simulink model "hw481pendulum"  (Simulink 7.0)
settings: Solver=ode45  StartTime=0.0  StopTime=20  FixedStep=Tsample  RelTol=1e-5
settings Model: Creator=Kostas Tsakalis  LastModifiedBy=KST  ExtModeArmWhenConnect=off  BufferReuse=off
settings DataIOCC: LimitDataPoints=off  SaveState=on  OutputSaveName=theta  SignalLoggingName=sigsOut
settings OptimizationCC: BlockReduction=off  OptimizeBlockIOStorage=off  BufferReuse=off  EnforceIntegerDowncast=off  ExpressionFolding=off  FoldNonRolledExpr=off  LocalBlockOutputs=off
settings DebuggingCC: SaveWithParameterizedLinksMsg=none  SignalResolutionControl=TryResolveAllWithWarning  SolverPrmCheckMsg=none  MultiTaskDSMMsg=warning  MultiTaskCondExecSysMsg=none  StrictBusMsg=None
settings HardwareCC: TargetEndianess=LittleEndian  TargetHWDeviceType=MATLAB Host  ProdEqTarget=off
settings RTWCC: SystemTargetFile=xpctarget.tlc  TemplateMakefile=xpc_default_tmf  Description=xPC Target  ProcessScript=xpctarget_make_rtw_hook  IncludeERTFirstTime=on
settings xpcTargetCC: TargetFcnLib=ansi_tfl_tmw.mat  GenFloatMathFcnCalls=ANSI_C  CompOptLevelCompliant=off  PortableWordSizes=off

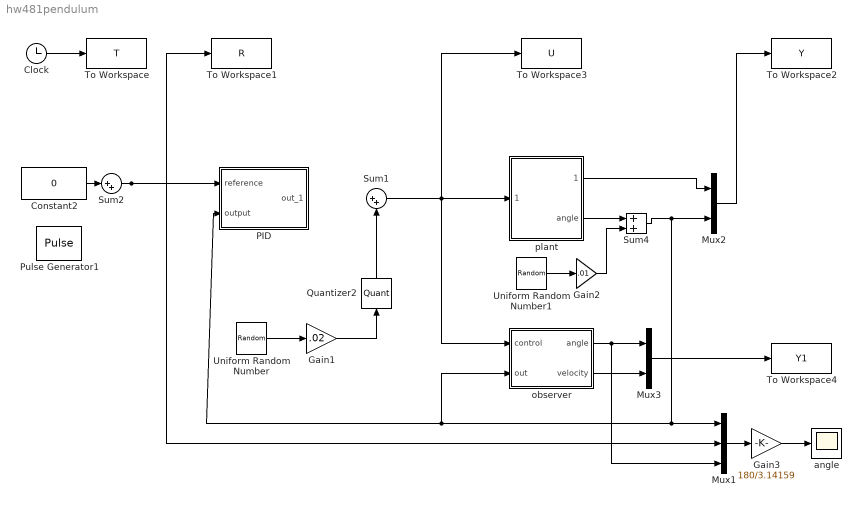
== system hw481pendulum ==
  Clock : Clock
      settings: Decimation=10
  Constant2 : Constant  Value=0  OutDataType=sfix(16)  OutScaling=2^0
  Gain1 : Gain  Gain=.02  ParameterDataType=sfix(16)  ParameterScaling=2^0  OutDataType=sfix(16)  OutScaling=2^0  SaturateOnIntegerOverflow=on
  Gain2 : Gain  Gain=.01  ParameterDataType=sfix(16)  ParameterScaling=2^0  OutDataType=sfix(16)  OutScaling=2^0  SaturateOnIntegerOverflow=on
  Gain3 : Gain  Gain=180/3.14159  ParameterDataType=sfix(16)  ParameterScaling=2^0  OutDataType=sfix(16)  OutScaling=2^0  SaturateOnIntegerOverflow=on
  Mux1 : Mux  Inputs=3
  Mux2 : Mux  Inputs=2
  Mux3 : Mux  Inputs=2
  PID : Subsystem
  Pulse Generator1 : DiscretePulseGenerator  PulseType=Time based  Amplitude=.2  Period=4  PulseWidth=50  PhaseDelay=1
  Quantizer2 : Quantizer  Orientation=up  QuantizationInterval=2/(2^10)
  Sum1 : Sum  Inputs=|++  OutDataType=sfix(16)  OutScaling=2^0  SaturateOnIntegerOverflow=on
  Sum2 : Sum  Inputs=|++  OutDataType=sfix(16)  OutScaling=2^0  SaturateOnIntegerOverflow=on
  Sum4 : Sum  Inputs=2  OutDataType=sfix(16)  OutScaling=2^0  SaturateOnIntegerOverflow=on
  To Workspace : ToWorkspace  VariableName=T  SampleTime=.01  SaveFormat=Array
  To Workspace1 : ToWorkspace  VariableName=R  SampleTime=.01  SaveFormat=Array
  To Workspace2 : ToWorkspace  VariableName=Y  SampleTime=.01  SaveFormat=Array
  To Workspace3 : ToWorkspace  VariableName=U  SampleTime=.01  SaveFormat=Array
  To Workspace4 : ToWorkspace  VariableName=Y1  SampleTime=.01  SaveFormat=Array
  Uniform Random Number : UniformRandomNumber  SampleTime=.1
  Uniform Random Number1 : UniformRandomNumber  SampleTime=.01
  angle : Scope
      settings: TickLabels=on  TimeRange=20  YMax=15  DataFormat=Array  MaxDataPoints=10000
  observer : Subsystem
  plant : Subsystem  mask{mass=0.2, length=0.5, friction=0, quant=360/(2^12), Sa=1, inquant=2/(2^10), IC=[0 0]}
      mask prompts: quant "quantization"; Sa "saturation (+/-)"; inquant "input quantization"; IC "Initial Conditions (2x1)"
      mask Display: disp('Pendulum \n model')
  wires:
  Constant2/1 -> Sum2/1
  Sum2/1 -> Mux1/2, To Workspace1/1, PID/1(reference)
  plant/2(angle) -> Sum4/1
  Gain3/1 -> angle/1
  Mux1/1 -> Gain3/1
  Clock/1 -> To Workspace/1
  Mux2/1 -> To Workspace2/1
  plant/1(velocity) -> Mux2/1
  Sum1/1 -> plant/1(control), To Workspace3/1, observer/1(control)
  Uniform Random Number/1 -> Gain1/1
  observer/1(angle) -> Mux3/1, Mux1/3
  observer/2(velocity) -> Mux3/2
  Mux3/1 -> To Workspace4/1
  Sum4/1 -> Mux1/1, PID/2(output), observer/2(out), Mux2/2
  Uniform Random Number1/1 -> Gain2/1
  Gain1/1 -> Quantizer2/1
  Quantizer2/1 -> Sum1/2
  Gain2/1 -> Sum4/2

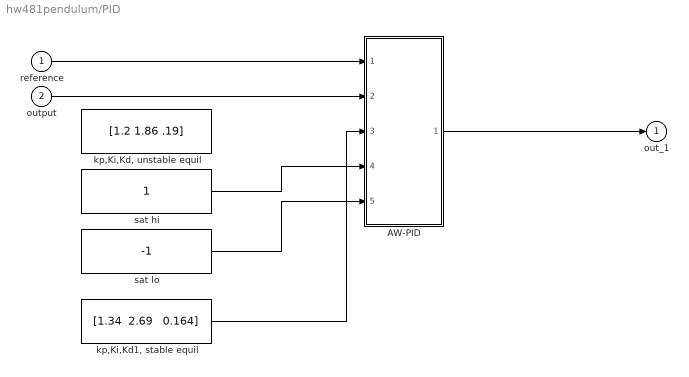
== system hw481pendulum/PID ==
  reference : Inport  OutDataType=sfix(16)  OutScaling=2^0
  output : Inport  Port=2  OutDataType=sfix(16)  OutScaling=2^0
  "AW-PID " : Subsystem  mask(Anti-windup PID ){tau=.005, DT=0.01}
      mask prompts: tau "Pseudo-derivative filter time constant (tustin)"; DT "Reference prefilter [num,den] time constants"
      mask help: Discrete PID with Anti-windup and prefilter
      mask init:
      | t_z=@2(1);t_p=@2(2);
      mask Display: disp('Adaptive\n AW-PID\n+filter')
  "kp,Ki,Kd, unstable equil" : Constant  Value=[1.2 1.86 .19]  OutDataType=sfix(16)  OutScaling=2^0  SampleTime=.01
  "kp,Ki,Kd1, stable equil" : Constant  Value="[1.34  2.69   0.164]"  OutDataType=sfix(16)  OutScaling=2^0  SampleTime=.01
  sat hi : Constant  OutDataType=sfix(16)  OutScaling=2^0
  sat lo : Constant  Value=-1  OutDataType=sfix(16)  OutScaling=2^0
  out_1 : Outport  InitialOutput=0
  wires:
  sat lo/1 -> "AW-PID "/5(input constraint lo)
  sat hi/1 -> "AW-PID "/4(input constraint hi)
  output/1 -> "AW-PID "/2(System Output)
  "AW-PID "/1(Input to system) -> out_1/1
  reference/1 -> "AW-PID "/1(Set point)
  "kp,Ki,Kd1, stable equil"/1 -> "AW-PID "/3(parameters)

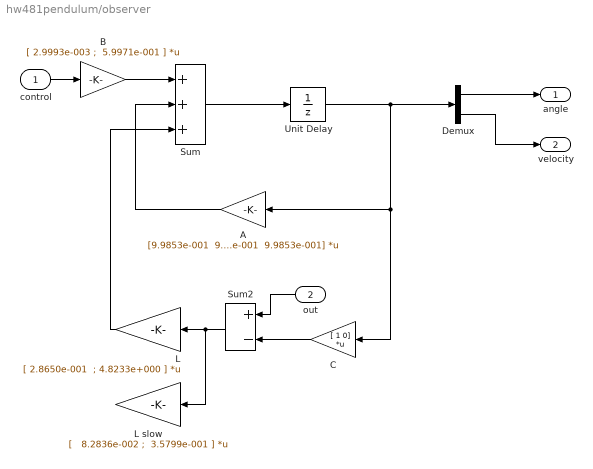
== system hw481pendulum/observer ==
  control : Inport  OutDataType=sfix(16)  OutScaling=2^0
  out : Inport  Orientation=left  Port=2  OutDataType=sfix(16)  OutScaling=2^0
  A : Gain  Orientation=left  Gain=|  Multiplication=Matrix(K*u)  ParameterDataType=sfix(16)  ParameterScaling=2^0  OutDataType=sfix(16)  OutScaling=2^0  SaturateOnIntegerOverflow=on
      | [9.9853e-001  9.9951e-003
      | ; -2.9416e-001  9.9853e-001]
  B : Gain  Gain=|  Multiplication=Matrix(K*u)  ParameterDataType=sfix(16)  ParameterScaling=2^0  OutDataType=sfix(16)  OutScaling=2^0  SaturateOnIntegerOverflow=on
      | [ 2.9993e-003;  5.9971e-001
      | ]
  C : Gain  Orientation=left  Gain="[  1     0]"  Multiplication=Matrix(K*u)  ParameterDataType=sfix(16)  ParameterScaling=2^0  OutDataType=sfix(16)  OutScaling=2^0  SaturateOnIntegerOverflow=on
  Demux : Demux  Outputs=2
  L : Gain  Orientation=left  Gain=|  Multiplication=Matrix(K*u)  ParameterDataType=sfix(16)  ParameterScaling=2^0  OutDataType=sfix(16)  OutScaling=2^0  SaturateOnIntegerOverflow=on
      | [ 2.8650e-001
      |  ; 4.8233e+000
      | ]
  L slow : Gain  Orientation=left  Gain=|  Multiplication=Matrix(K*u)  ParameterDataType=sfix(16)  ParameterScaling=2^0  OutDataType=sfix(16)  OutScaling=2^0  SaturateOnIntegerOverflow=on
      | [   8.2836e-002
      | ;  3.5799e-001
      | ]
  Sum : Sum  Inputs=+++  OutDataType=sfix(16)  OutScaling=2^0  SaturateOnIntegerOverflow=on  InputSameDT=on
  Sum2 : Sum  Orientation=left  Inputs=+-  OutDataType=sfix(16)  OutScaling=2^0  SaturateOnIntegerOverflow=on  InputSameDT=on
  Unit Delay : UnitDelay  SampleTime=.01
  angle : Outport  InitialOutput=0
  velocity : Outport  Port=2  InitialOutput=0
  wires:
  Sum2/1 -> L/1, L slow/1
  out/1 -> Sum2/1
  control/1 -> B/1
  Sum/1 -> Unit Delay/1
  Unit Delay/1 -> Demux/1, A/1, C/1
  Demux/1 -> angle/1
  Demux/2 -> velocity/1
  A/1 -> Sum/2
  B/1 -> Sum/1
  C/1 -> Sum2/2
  L/1 -> Sum/3

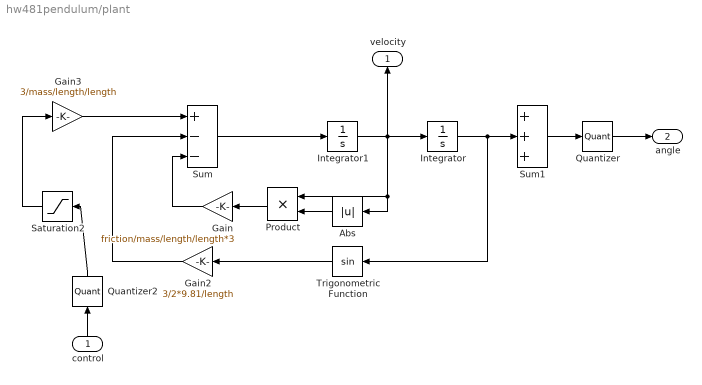
== system hw481pendulum/plant ==
  control : Inport  Orientation=up  OutDataType=sfix(16)  OutScaling=2^0
  Abs : Abs  Orientation=left  OutDataType=sfix(16)  OutScaling=2^0
  Gain : Gain  Orientation=left  Gain=friction/mass/length/length*3  ParameterDataType=sfix(16)  ParameterScaling=2^0  OutDataType=sfix(16)  OutScaling=2^0  SaturateOnIntegerOverflow=on
  Gain2 : Gain  Orientation=left  Gain=3/2*9.81/length  ParameterDataType=sfix(16)  ParameterScaling=2^0  OutDataType=sfix(16)  OutScaling=2^0  SaturateOnIntegerOverflow=on
  Gain3 : Gain  Gain=3/mass/length/length  ParameterDataType=sfix(16)  ParameterScaling=2^0  OutDataType=sfix(16)  OutScaling=2^0  SaturateOnIntegerOverflow=on
  Integrator : Integrator  InitialCondition=IC(1)
  Integrator1 : Integrator  InitialCondition=IC(2)
  Product : Product  Orientation=left  OutDataType=sfix(16)  OutScaling=2^0  RndMeth=Zero
  Quantizer : Quantizer  QuantizationInterval=quant*pi/180
  Quantizer2 : Quantizer  Orientation=up  QuantizationInterval=inquant
  Saturation2 : Saturate  Orientation=left  UpperLimit=Sa  LowerLimit=-Sa
  Sum : Sum  Inputs=+--  OutDataType=sfix(16)  OutScaling=2^0  SaturateOnIntegerOverflow=on  InputSameDT=on
  Sum1 : Sum  Inputs=+++  OutDataType=sfix(16)  OutScaling=2^0  SaturateOnIntegerOverflow=on  InputSameDT=on
  Trigonometric Function : Trigonometry  Orientation=left
  velocity : Outport  Orientation=up  InitialOutput=0
  angle : Outport  Port=2  InitialOutput=0
  wires:
  Quantizer/1 -> angle/1
  Sum1/1 -> Quantizer/1
  control/1 -> Quantizer2/1
  Gain3/1 -> Sum/1
  Gain2/1 -> Sum/2
  Integrator/1 -> Sum1/2, Trigonometric Function/1
  Gain/1 -> Sum/3
  Integrator1/1 -> Integrator/1, velocity/1, Product/1, Abs/1
  Saturation2/1 -> Gain3/1
  Trigonometric Function/1 -> Gain2/1
  Sum/1 -> Integrator1/1
  Product/1 -> Gain/1
  Abs/1 -> Product/2
  Quantizer2/1 -> Saturation2/1

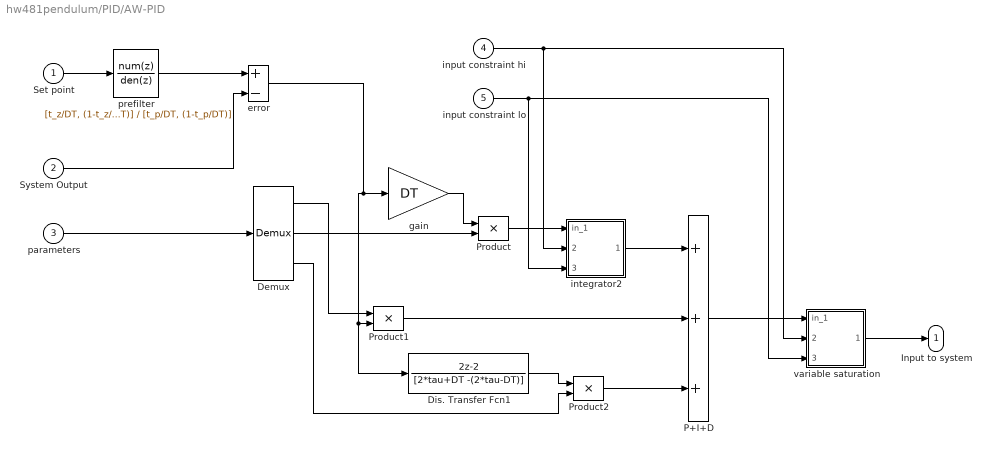
== system hw481pendulum/PID/AW-PID  ==
  Set point : Inport  OutDataType=sfix(16)  OutScaling=2^0
  System Output : Inport  Port=2  OutDataType=sfix(16)  OutScaling=2^0
  parameters : Inport  Port=3  OutDataType=sfix(16)  OutScaling=2^0
  input constraint hi : Inport  Port=4  OutDataType=sfix(16)  OutScaling=2^0
  input constraint lo : Inport  Port=5  OutDataType=sfix(16)  OutScaling=2^0
  Demux : Demux  Outputs=3
  Dis. Transfer Fcn1 : DiscreteTransferFcn  Numerator=[2 -2]  Denominator=[2*tau+DT -(2*tau-DT)]  SampleTime=DT
  P+I+D : Sum  Inputs=+++  OutDataType=sfix(16)  OutScaling=2^0  SaturateOnIntegerOverflow=on  InputSameDT=on
  Product : Product  OutDataType=sfix(16)  OutScaling=2^0  SaturateOnIntegerOverflow=on  InputSameDT=on
  Product1 : Product  OutDataType=sfix(16)  OutScaling=2^0  SaturateOnIntegerOverflow=on  InputSameDT=on
  Product2 : Product  OutDataType=sfix(16)  OutScaling=2^0  SaturateOnIntegerOverflow=on  InputSameDT=on
  error : Sum  Inputs=+-  OutDataType=sfix(16)  OutScaling=2^0  SaturateOnIntegerOverflow=on  InputSameDT=on
  gain : Gain  Gain=DT  ParameterDataType=sfix(16)  ParameterScaling=2^0  OutDataType=sfix(16)  OutScaling=2^0  SaturateOnIntegerOverflow=on
  integrator2 : Subsystem  mask(Anti windup intgrator){DT=DT}
      mask prompts: DT "sampling time"
      mask help: Integral with anti-windup
      mask Display: disp('DT-I-AW')
  prefilter : DiscreteTransferFcn  Numerator=[t_z/DT, (1-t_z/DT)]  Denominator=[t_p/DT, (1-t_p/DT)]  SampleTime=DT
  variable saturation : Subsystem  mask(Anti windup intgrator){DT=DT}
      mask prompts: DT "sampling time"
      mask help: Integral with anti-windup
      mask Display: disp('DT-I-AW')
  Input to system : Outport  InitialOutput=0
  wires:
  input constraint hi/1 -> variable saturation/2(umax), integrator2/2(umax)
  input constraint lo/1 -> variable saturation/3(umin), integrator2/3(umin)
  variable saturation/1(out_1) -> Input to system/1
  System Output/1 -> error/2
  Demux/3 -> Product2/2
  Dis. Transfer Fcn1/1 -> Product2/1
  Product2/1 -> P+I+D/3
  Demux/2 -> Product/2
  Demux/1 -> Product1/1
  gain/1 -> Product/1
  Product/1 -> integrator2/1(in_1)
  P+I+D/1 -> variable saturation/1(in_1)
  integrator2/1(out_1) -> P+I+D/1
  parameters/1 -> Demux/1
  Set point/1 -> prefilter/1
  Product1/1 -> P+I+D/2
  error/1 -> gain/1, Product1/2, Dis. Transfer Fcn1/1
  prefilter/1 -> error/1

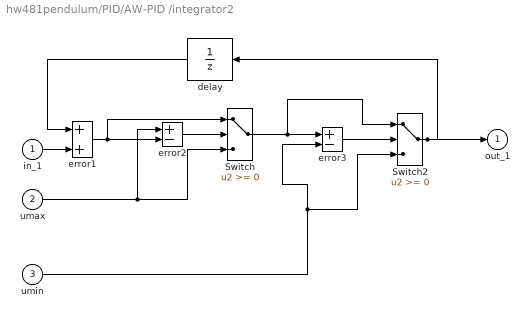
== system hw481pendulum/PID/AW-PID /integrator2 ==
  in_1 : Inport  OutDataType=sfix(16)  OutScaling=2^0
  umax : Inport  Port=2  OutDataType=sfix(16)  OutScaling=2^0
  umin : Inport  Port=3  OutDataType=sfix(16)  OutScaling=2^0
  Switch : Switch  SaturateOnIntegerOverflow=on  InputSameDT=on
  Switch2 : Switch  SaturateOnIntegerOverflow=on  InputSameDT=on
  delay : DiscreteTransferFcn  Orientation=left  Denominator=[1 0]  SampleTime=DT
  error1 : Sum  OutDataType=sfix(16)  OutScaling=2^0  SaturateOnIntegerOverflow=on  InputSameDT=on
  error2 : Sum  Inputs=+-  OutDataType=sfix(16)  OutScaling=2^0  SaturateOnIntegerOverflow=on  InputSameDT=on
  error3 : Sum  Inputs=+-  OutDataType=sfix(16)  OutScaling=2^0  SaturateOnIntegerOverflow=on  InputSameDT=on
  out_1 : Outport  InitialOutput=0
  wires:
  in_1/1 -> error1/2
  Switch2/1 -> out_1/1, delay/1
  Switch/1 -> Switch2/1, error3/1
  error1/1 -> Switch/1, error2/2
  umax/1 -> Switch/3, error2/1
  umin/1 -> Switch2/3, error3/2
  error3/1 -> Switch2/2
  error2/1 -> Switch/2
  delay/1 -> error1/1

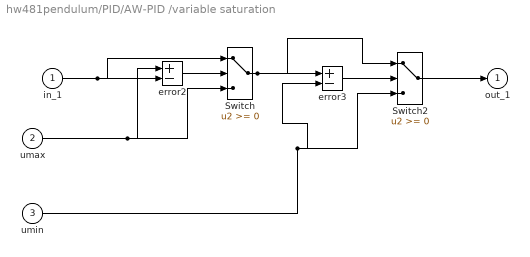
== system hw481pendulum/PID/AW-PID /variable saturation ==
  in_1 : Inport  OutDataType=sfix(16)  OutScaling=2^0
  umax : Inport  Port=2  OutDataType=sfix(16)  OutScaling=2^0
  umin : Inport  Port=3  OutDataType=sfix(16)  OutScaling=2^0
  Switch : Switch  SaturateOnIntegerOverflow=on  InputSameDT=on
  Switch2 : Switch  SaturateOnIntegerOverflow=on  InputSameDT=on
  error2 : Sum  Inputs=+-  OutDataType=sfix(16)  OutScaling=2^0  SaturateOnIntegerOverflow=on  InputSameDT=on
  error3 : Sum  Inputs=+-  OutDataType=sfix(16)  OutScaling=2^0  SaturateOnIntegerOverflow=on  InputSameDT=on
  out_1 : Outport  InitialOutput=0
  wires:
  error2/1 -> Switch/2
  error3/1 -> Switch2/2
  umin/1 -> error3/2, Switch2/3
  umax/1 -> error2/1, Switch/3
  Switch/1 -> error3/1, Switch2/1
  Switch2/1 -> out_1/1
  in_1/1 -> error2/2, Switch/1
